simulink library "allocation_lib"  (R2018b)
settings: Solver=VariableStepAuto  StartTime=0.0  StopTime=10.0  RelTol=1e-3
undefined symbols (not defined in the file or in its folder): fswParams
settings Model: Creator=colem  LastModifiedBy=colem

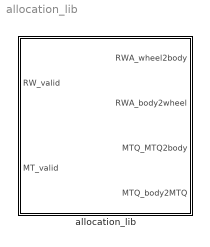
== system allocation_lib ==
  allocation_lib : Subsystem

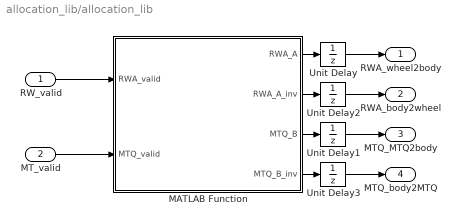
== system allocation_lib/allocation_lib ==
  RW_valid : Inport
  MT_valid : Inport  Port=2
  MATLAB Function : MATLAB Function  TreatAsAtomicUnit=on
  Unit Delay : UnitDelay  InitialCondition=fswParams.allocator.A  SampleTime=-1
  Unit Delay1 : UnitDelay  InitialCondition=[1 1 1 1 1]  SampleTime=-1
  Unit Delay2 : UnitDelay  InitialCondition=fswParams.allocator.A_inv  SampleTime=-1
  Unit Delay3 : UnitDelay  InitialCondition=fswParams.allocator.A_inv  SampleTime=-1
  RWA_wheel2body : Outport
  RWA_body2wheel : Outport  Port=2
  MTQ_MTQ2body : Outport  Port=3
  MTQ_body2MTQ : Outport  Port=4
  wires:
  Unit Delay/1 -> RWA_wheel2body/1
  RW_valid/1 -> MATLAB Function/1(RWA_valid)
  MATLAB Function/1(RWA_A) -> Unit Delay/1
  MT_valid/1 -> MATLAB Function/2(MTQ_valid)
  MATLAB Function/3(MTQ_B) -> Unit Delay1/1
  Unit Delay1/1 -> MTQ_MTQ2body/1
  Unit Delay2/1 -> RWA_body2wheel/1
  MATLAB Function/2(RWA_A_inv) -> Unit Delay2/1
  MATLAB Function/4(MTQ_B_inv) -> Unit Delay3/1
  Unit Delay3/1 -> MTQ_body2MTQ/1

== matlab function allocation_lib/MATLAB Function ==
  data: RWA_valid input; RWA_A output; RWA_A_inv output; MTQ_valid input; MTQ_B output; MTQ_B_inv output
% Logic for selecting the gnc allocation scheme
%
% Author: Cole Morgan 
%
% 



function [RWA_A, RWA_A_inv, MTQ_B, MTQ_B_inv]  = allocation_logic(RWA_valid, MTQ_valid)

%GNC_ALLOCATION_LOGIC    GNC Allocation Selector
%
% Chooses allocation scheme based on actuator validity.
%
%   RW_A = The mapping from tau_c (the 4x1 wheel-frame torque command)
%       to u_c (the 3x1 vector of body-frame commands).
%       This is a 3x4 mapping. 4 wheels composed into 3 principal
%       directions.
%   RW_A_inv = The mapping from u_c (the 3x1 total body-frame torque command)
%       to tau_c (the 4x1 vector of comanded torques to each individual wheel).
%       This is a 4x3 mapping. 3 directions distributed into 4 wheels.
%   MT_B = A vector containing the necessary gain to each MT. Recall, the MTs are
%       alligned with the body axes. Therefore a torque commanded in the
%       body frame passes "straight through", only to be gained depending
%       on availability or direction. The notation is: [+x -x +y -y +z].
%       An example is [1 -1 0 -1 1] indicating that the +y-face MT is
%       unoperational.
%
% ----- INPUTS -----
%
% 1. RW_valid - a 1x4 vector containing the availability of the 4 RWA wheels.
%       An example is [1 1 0 1], which indicates that wheel_3 is
%       unoperational. The RW_Phi mapping changes accordingly.
%
% 2. MT_valid - a 1x5 vector containing the availability of the 5 Magnetorquers.
%       An example is [1 1 0 1 1], which indicates that +y-face MT is
%       unoperational. The MT_B mapping (gain) changes accordingly.
%
% -------------------------------------------------------------------------------

% Wheel to body frame is based only on available wheels.
RWA_A = fswParams.allocator.RWA_A*diag([RWA_valid]);

% MTQ to body is based only on availabe MTQs.
MTQ_B = fswParams.allocator.MTQ_B*diag([MTQ_valid]);

% Assume all actuators are availabe for inverse before checking.
RWA_A_inv     = fswParams.allocator.RWA_A_inv;
MTQ_B_inv     = fswParams.allocator.MTQ_B_inv;

%check how many RWA wheels are dead
num_dead_RWA = sum(RWA_valid == 0);
if (num_dead_RWA > 0 && num_dead_RWA < 2)
    
    % zeros the column of dead wheel from A
    temp = fswParams.allocator.RWA_A*diag([RWA_valid]);
    RWA_A_inv = temp'/(temp*temp');
    % This method does not work if two wheels are dead
    % becuase two vectors cannot span R3. Then RWA_A_inv
    % will be NaN. inv of singular matrix.
    
%     if (RW_valid == [0 1 1 1])
%         RW_Phi = fswParams.allocator.Phi_1;
%     elseif (RW_valid == [1 0 1 1])
%         RW_Phi = fswParams.allocator.Phi_2;
%     elseif (RW_valid == [1 1 0 1])
%         RW_Phi = fswParams.allocator.Phi_3;
%     elseif (RW_valid == [1 1 1 0])
%         RW_Phi = fswParams.allocator.Phi_4;
%     end
% end
% % notice that if two wheels are dead, the default RWA_A_inv will still
% % be used. This is a potential problem.

elseif(num_dead_RWA >= 2)
    
    % Uses the original RWA_A_inv but zeros the dead columns of RWA_A_inv.
    % note this will not be an optimal RWA_A_inv, but it seems better than
    % doing nothing.
    RWA_A_inv = diag([RWA_valid])*RWA_A_inv;
end


%%%% MTQ %%%%

% check how many MTQ are dead
num_dead_MTQ = sum(MTQ_valid == 0);

if (num_dead_MTQ > 0)
    
    % now check to see if all MTQ(s) are dead in the any direction.
    % this will ruin the possibility if determining MTQ_B_inv.
    % This if condition is satisfied in the bad scenario that say both
    % x-facing or both y-facing or the z MTQ(s) are dead.
    if ((~(MTQ_valid(1) || MTQ_valid(2)) || ~(MTQ_valid(3) || MTQ_valid(4)) || ~MTQ_valid(5))) 
        % Uses the original MTQ_B_inv but zeros the dead columns of MTQ_B_inv.
        % note this will not be an optimal MTQ_B_inv, but it seems better than
        % doing nothing.
        MTQ_B_inv = diag([MTQ_valid])*MTQ_B_inv;
    else
        % zeros the column of dead MTQ from B
        temp = fswParams.allocator.MTQ_B*diag([MTQ_valid]);
        MTQ_B_inv = temp'/(temp*temp');
        % This method does not work if two MTQs are dead from the
        % same face becuase two vectors cannot span R3. Then MTQ_B_inv
        % will be NaN. inv of singular matrix.
    end
end
